simulink model "model_astolfi"  (R2014b)
settings: Solver=ode23  StartTime=0.0  StopTime=15.0  RelTol=1e-10
values from neighbouring files (symbols this model uses):
  k = 1    [astolfi.m]    (also in monocykl.m)
  p2 = -7    [astolfi.m]    (also in monocykl.m)
  p3 = 12    [astolfi.m]    (also in monocykl.m)
settings Model: Creator=lab1.5  LastModifiedBy=Dawid Perdek

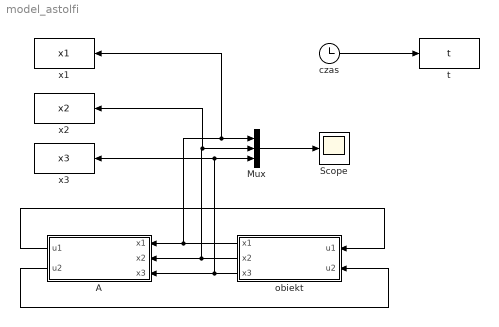
== system model_astolfi ==
  A : Subsystem
  Mux : Mux  Inputs=3
  Scope : Scope
  czas : Clock
  obiekt : Subsystem
  t : ToWorkspace  VariableName=t  SampleTime=-1
  x1 : ToWorkspace  VariableName=x1  SampleTime=-1
  x2 : ToWorkspace  VariableName=x2  SampleTime=-1
  x3 : ToWorkspace  VariableName=x3  SampleTime=-1
  wires:
  A/1(u1) -> obiekt/1(u1)
  A/2(u2) -> obiekt/2(u2)
  obiekt/1(x1) -> x1/1, Mux/1, A/1(x1)
  obiekt/2(x2) -> A/2(x2), x2/1, Mux/2
  obiekt/3(x3) -> A/3(x3), x3/1, Mux/3
  Mux/1 -> Scope/1
  czas/1 -> t/1

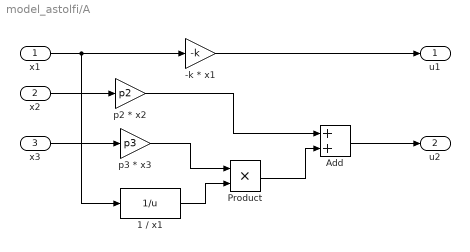
== system model_astolfi/A ==
  x1 : Inport
  x2 : Inport  Port=2
  x3 : Inport  Port=3
  -k * x1 : Gain  Gain=-k
  1 / x1 : Fcn  Expr=1/u
  Add : Sum
  Product : Product
  p2 * x2 : Gain  Gain=p2
  p3 * x3 : Gain  Gain=p3
  u1 : Outport
  u2 : Outport  Port=2
  wires:
  p3 * x3/1 -> Product/1
  1 / x1/1 -> Product/2
  x1/1 -> 1 / x1/1, -k * x1/1
  x2/1 -> p2 * x2/1
  -k * x1/1 -> u1/1
  p2 * x2/1 -> Add/1
  x3/1 -> p3 * x3/1
  Add/1 -> u2/1
  Product/1 -> Add/2

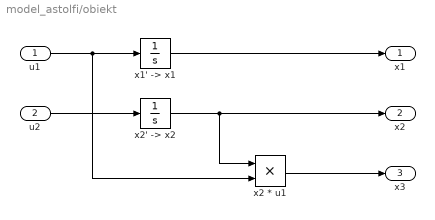
== system model_astolfi/obiekt ==
  u1 : Inport
  u2 : Inport  Port=2
  "x1' -> x1" : Integrator  InitialCondition=1
  x2 * u1 : Product
  "x2' -> x2" : Integrator  InitialCondition=2
  x1 : Outport
  x2 : Outport  Port=2
  x3 : Outport  Port=3
  wires:
  u1/1 -> x2 * u1/2, "x1' -> x1"/1
  "x1' -> x1"/1 -> x1/1
  u2/1 -> "x2' -> x2"/1
  "x2' -> x2"/1 -> x2 * u1/1, x2/1
  x2 * u1/1 -> x3/1
